simulink model "deadbeat_running_control"  (R2016b)
settings: configuration reference "Configuration1khz" (kept outside this file)
undefined symbols (not defined in the file or in its folder): A_kalman_no_position, A_kalman_transverse, A_kalman_vertical, A_lpf_accelerometer, A_lpf_contact, A_lpf_imu, A_lpf_lateral_angle, B1_lpf_accelerometer, B1_lpf_contact, B1_lpf_imu, B1_lpf_lateral_angle, B2_lpf_accelerometer, B2_lpf_contact, B2_lpf_imu, B2_lpf_lateral_angle, B_dx_versus_x0, B_kalman_no_position, B_kalman_transverse, B_kalman_vertical, backwards_K_sag_of_t, backwards_P_sag_of_t, C_kalman_no_position, C_kalman_transverse, C_kalman_vertical, com_leg_motor, com_torso, contact_threshold, d_ankle_to_foot, d_vertical_com, desired_com_forward_velocity, desired_com_lateral_velocity, desired_standing_torso_pitch, desired_standing_torso_roll, desired_standing_z, desired_torso_pitch, desired_torso_roll, DiscIntNeverNeededParam, Discrete, enable_bouncing, fdesignblkfcn, flight_duration, forward_dx_of_dxstar, forward_x_of_dxstar, g, gcbh, HIP_MTR_MAX_CONT_TORQUE, HIP_MTR_MAX_TORQUE, i_leg_motor, i_robot, i_torso, initial_dx_estimate, initial_dx_takeoff_history, initial_dx_touchdown_history, initial_dy_estimate, initial_dy_takeoff_history, initial_dy_touchdown_history, initial_dz_estimate, initial_leg_selection, initial_target_dx_history, initial_target_dy_history ... (+80)
libraries: simulink x22, ctrlSharedLib x4, dsparch4 x2
(part 4 of 7)

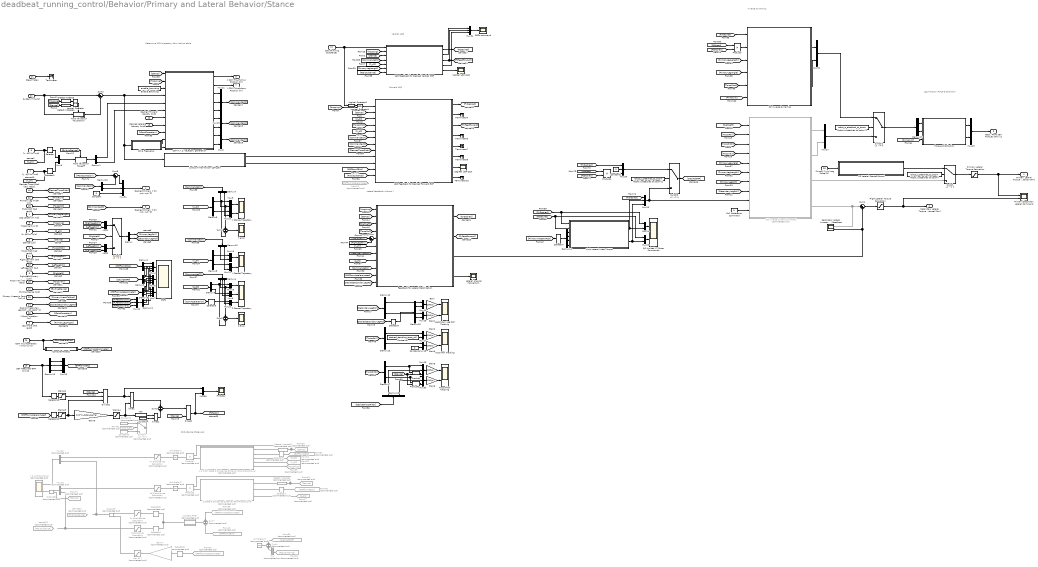
== system deadbeat_running_control/Behavior/Primary and Lateral Behavior/Stance ==
  note: Leg Torque / Force
      | Distribution
  note: Disturbance Observers
  note: Determine COM trajectory
      | from lookup table
  note: Forward LQR
  note: Inverse Dynamics
  note: Lateral feedback without Y
  note: Vertical LQR
  Leg Length [m m/s] : Inport
  Torso Pitch [rad rad/s] : Inport  Port=2
  Stance [1/0] : Inport  Port=3
  Leg Angle [rad rad/s] : Inport  Port=4
  Right/Left Primary [1/0] : Inport  Port=5
  "[x, dx] [m, m/s]" : Inport  Port=6
  "[y, dy] [m, m/s]" : Inport  Port=7
  "[z, dz] [m, m/s]" : Inport  Port=8
  Hopping [1 or 0] : Inport  Port=9
  SEA Measured GRF [N N N] : Inport  Port=10
  Steps Taken : Inport  Port=11
  Desired Forward Velocity [m/s] : Inport  Port=12
  Desired Lateral Velocity [m/s] : Inport  Port=13
  Right Leg Roll [rad rad/s] : Inport  Port=14
  Left Leg Roll [rad rad/s] : Inport  Port=15
  Torso Yaw [rad rad/s] : Inport  Port=16
  Exiting Stance [1/0] : Inport  Port=17
  "Desired Torso Pitch [rad, rad/s]" : Inport  Port=18
  Torso Roll [rad rad/s] : Inport  Port=19
  COM XYZ Acceleration [m/s^2] x3 : Inport  Port=20
  System Time [s] : Inport  Port=21
  Primary Leg Width [m] : Inport  Port=22
  Primary Knees to Foot [m] x6 : Inport  Port=23
  Desired Secondary Leg Roll [rad rad/s rad/s^2] : Inport  Port=24
  Primary Axial Leg Force [N] : Inport  Port=25
  X Foot Correction [m[ : Inport  Port=26
  Stop Running [true/false] : Inport  Port=27
  2D Inverse Dynamics : Subsystem
  2D Lateral Stance Control : MATLAB Function  TreatAsAtomicUnit=on
  3D Inverse Dynamics yawed : MATLAB Function  Commented=on  TreatAsAtomicUnit=on
  COM X,Y,Z  trajectory generation : MATLAB Function  TreatAsAtomicUnit=on
  Chirp Frequency : Subsystem
  Clamp2 : Saturate  UpperLimit=inf  LowerLimit=0
      settings: AttributesFormatString=Top: %<UpperLimit>\nBottom: %<LowerLimit>
  Clamp3 : Saturate  UpperLimit=inf  LowerLimit=1
      settings: AttributesFormatString=Top: %<UpperLimit>\nBottom: %<LowerLimit>
  Clamp4 : Saturate  UpperLimit=1  LowerLimit=0
      settings: AttributesFormatString=Top: %<UpperLimit>\nBottom: %<LowerLimit>
  Compute Forces1 : Subsystem
  Constant : Constant  Value=0
  Constant1 : Constant  Value=0
  Constant2 : Constant  Commented=on
  Constant3 : Constant  Value=desired_standing_torso_roll
  Constant4 : Constant  Value=0
  Constant5 : Constant  Commented=on  Value=0.87
  Constant6 : Constant
  Demux{,1,5,7..10,12..13,15,17..20} (14 alike) : Demux  Outputs=2
  Demux{2..4,6,11,16} (6 alike) : Demux  Outputs=3
  Demux14 : Demux
  Detect Increase : simulink/Logic and Bit Operations/Detect Increase  vinit=0.0  InputProcessing=Inherited  OutDataTypeStr=boolean
  Detect Increase1 : simulink/Logic and Bit Operations/Detect Increase  vinit=0.0  InputProcessing=Inherited  OutDataTypeStr=boolean
  Detect Increase2 : simulink/Logic and Bit Operations/Detect Increase  Commented=on  vinit=0.0  InputProcessing=Inherited  OutDataTypeStr=boolean
  Detect Increase3 : simulink/Logic and Bit Operations/Detect Increase  Commented=on  vinit=0.0  InputProcessing=Inherited  OutDataTypeStr=boolean
  "Disturbance Saturation " : Saturate  Commented=on  UpperLimit=100  LowerLimit=-100
      settings: AttributesFormatString=Top: %<UpperLimit>\nBottom: %<LowerLimit>
  Divide1 : Product  Inputs=**/
  Enable Bouncing : Constant  Value=enable_bouncing  SampleTime=sample_time
  Fcn : Fcn  Expr=1-u
  Feedback for Lateral Stabilization : MATLAB Function  TreatAsAtomicUnit=on
  Flight Lateral Torque Saturation : Saturate  UpperLimit=HIP_MTR_MAX_CONT_TORQUE  LowerLimit=-HIP_MTR_MAX_CONT_TORQUE
      settings: AttributesFormatString=Top: %<UpperLimit>\nBottom: %<LowerLimit>
  From10 : From  Commented=on  GotoTag=GRFfromAccelerometer
  From40 : From  Commented=on  GotoTag=GRFfromSEAs
  From47 : From  Commented=on  GotoTag=Z_dZ
  From48 : From  Commented=on  GotoTag=GRFfromSEAs
  From49 : From  Commented=on  GotoTag=Stance
  From50 : From  Commented=on  GotoTag=Stance
  From51 : From  Commented=on  GotoTag=GRFfromSEAs
  From52 : From  Commented=on  GotoTag=X_dX
  From53 : From  Commented=on  GotoTag=TorsoPitch
  From54 : From  Commented=on  GotoTag=Z_dZ
  From59 : From  Commented=on  GotoTag=GRFfromAccelerometer
  From61 : From  Commented=on  GotoTag=GRFfromAccelerometer
  From79 : From  Commented=on  GotoTag=Stance
  From80 : From  Commented=on  GotoTag=DesiredGRF
  From81 : From  Commented=on  GotoTag=FzDisturbance
  From82 : From  Commented=on  GotoTag=RightLeft
  Fx Disturbance Saturation : Saturate  Commented=on  UpperLimit=100  LowerLimit=-100
      settings: AttributesFormatString=Top: %<UpperLimit>\nBottom: %<LowerLimit>
  "Fx Disturbance Saturation " : Saturate  Commented=on  UpperLimit=30  LowerLimit=-30
      settings: AttributesFormatString=Top: %<UpperLimit>\nBottom: %<LowerLimit>
  Fz Disturbance Saturation : Saturate  Commented=on  UpperLimit=100  LowerLimit=-100
      settings: AttributesFormatString=Top: %<UpperLimit>\nBottom: %<LowerLimit>
  Fz Factor : Scope
  GRFs : Scope  NumInputPorts=3
  GRFz command : Scope
  Gain{,1..3,5..6} (6 alike) : Gain  Gain=180/pi
  Gain4 : Gain  Commented=on  Gain=2/(m_total_real*g)
  Gain8 : Gain  Gain=1/(2*m_total_real*g)
  Hold Values on Takeoff : Subsystem
  Hold Values on Touchdown : Subsystem
  LQR Feedback for Desired Forward GRF : MATLAB Function  TreatAsAtomicUnit=on
  LQR Feedback for Desired Vertical GRF : MATLAB Function  TreatAsAtomicUnit=on
  Lateral Angular Momentum : Scope
  Limit Lateral Knee Torque : MATLAB Function  TreatAsAtomicUnit=on
  Logical Operator : Logic  Operator=OR  AllPortsSameDT=off  OutDataTypeStr=boolean
  Logical Operator1 : Logic  AllPortsSameDT=off  OutDataTypeStr=boolean
  Logical Operator2 : Logic  Operator=NOT  AllPortsSameDT=off  OutDataTypeStr=boolean
  Lookup finite horizon LQR gain : MATLAB Function  TreatAsAtomicUnit=on
  Lowpass Filter : Subsystem  Commented=on  DialogController=fdesignblkfcn  InitFcn=fdesignblkfcn(gcbh, {'InitFcn'});  mask(Lowpass Filter){}
      mask help: Design a lowpass filter
      settings: CopyFcn=fdesignblkfcn(gcbh, {'CopyFcn'});
      mask Help: helpview(mapfilelocation('dsp'), 'dsplowpassfilter');
      mask Display: disp('Lowpass')
  Max of 1 : Saturate  Commented=on  UpperLimit=1  LowerLimit=0
      settings: AttributesFormatString=Top: %<UpperLimit>\nBottom: %<LowerLimit>
  Mux : Mux  Commented=on  Inputs=3
  Mux{1..3,5,8..10,12..18,22..25,27,32,35,49} (22 alike) : Mux  Inputs=2
  Mux{11,21,26,28..31,33..34} (9 alike) : Mux  Inputs=3
  Mux19 : Mux  Commented=on  Inputs=2
  Mux20 : Mux  Commented=on  Inputs=2
  Mux4 : Mux
  Mux6 : Mux
  Mux7 : Mux
  Primary Lateral Torque Saturation : Saturate  UpperLimit=max_primary_lateral_stance_torque  LowerLimit=-max_primary_lateral_stance_torque
      settings: AttributesFormatString=Top: %<UpperLimit>\nBottom: %<LowerLimit>
  Primary/Secondary Lateral Command : Scope  NumInputPorts=2
  Product{,4,6..7} (4 alike) : Product
  Product{1..3,5} (4 alike) : Product  Commented=on
  QP Limited YZ Force Commands : Scope  NumInputPorts=2
  Robot is attached to boom? : Constant  Value=robot_is_attached_to_boom
  Robot is attached to boom?1 : Constant  Value=robot_is_attached_to_boom
  Robot is attached to boom?2 : Constant  Value=robot_is_attached_to_boom
  Roll Accleration Command : Constant  Value=0
  Sagittal LQR Cost : Scope
  Secondary Lateral Inverse Dynamics / Feedback : Scope  NumInputPorts=2
  Secondary Leg Roll Tracking : Scope  NumInputPorts=2
  Selector : Selector  InputPortWidth=2  IndexOptions=Index vector (dialog)  Indices=[2]  OutputSizes=1
  Selector1 : Selector  InputPortWidth=2  IndexOptions=Index vector (dialog)  Indices=[2]  OutputSizes=1
  Selector10 : Selector  InputPortWidth=3  IndexOptions=Index vector (dialog)  Indices=[3]  OutputSizes=1
  Selector11 : Selector  InputPortWidth=3  IndexOptions=Index vector (dialog)  Indices=[3]  OutputSizes=1
  Selector2 : Selector  Commented=on  InputPortWidth=3  IndexOptions=Index vector (dialog)  Indices=[3]  OutputSizes=1
  Selector3 : Selector  Commented=on  InputPortWidth=3  IndexOptions=Index vector (dialog)  Indices=[1]  OutputSizes=1
  Selector4 : Selector  Commented=on  InputPortWidth=3  IndexOptions=Index vector (dialog)  Indices=[3]  OutputSizes=1
  Selector5 : Selector  Commented=on  InputPortWidth=3  IndexOptions=Index vector (dialog)  Indices=[1]  OutputSizes=1
  Selector6 : Selector  InputPortWidth=3  IndexOptions=Index vector (dialog)  Indices=[3]  OutputSizes=1
  Selector7 : Selector  InputPortWidth=6  IndexOptions=Index vector (dialog)  Indices=[2 5 3 6]  OutputSizes=1
  Selector8 : Selector  Commented=on  InputPortWidth=3  IndexOptions=Index vector (dialog)  Indices=[3]  OutputSizes=1
  Selector9 : Selector  InputPortWidth=3  IndexOptions=Index vector (dialog)  Indices=[1 2]  OutputSizes=1
  Sum : Sum  Inputs=|+-
  Sum1 : Sum  Commented=on
  Sum2 : Sum  Inputs=|+-
  Sum3 : Sum  Inputs=+|+
  Sum4 : Sum  Inputs=|++
  Sum5 : Sum  Inputs=+-
  Sum6 : Sum  Inputs=+-
  Sum7 : Sum  Commented=on  Inputs=+-
  Sum8 : Sum  Inputs=|++
  Switch{,1..3} (4 alike) : Switch  Criteria=u2 ~= 0
  Switch4 : Switch  Commented=on  Criteria=u2 ~= 0
  Terminator{,4,6..8,10} (6 alike) : Terminator
  Torque Distribution : Subsystem
  Torso Pitch Tracking : Scope  NumInputPorts=2
  Torso Roll Tracking : Scope  NumInputPorts=2
  Unit Delay1 : UnitDelay  Commented=on  SampleTime=sample_time
  Unit Delay2 : UnitDelay  Commented=on  SampleTime=sample_time
  Unit Delay3 : UnitDelay  Commented=on  SampleTime=sample_time
  Vertical LQR Cost : Scope
  X & Pitch State Disturbance Observer Error-Proportional : MATLAB Function  Commented=on  TreatAsAtomicUnit=on
  X & Z Disturbance : Scope  Commented=on  NumInputPorts=2
  X Stance Trajectory : Scope  NumInputPorts=2
  X error : Scope
  Y Stance Trajectory : Scope  NumInputPorts=2
  Z Error : Scope
  Z Stance Trajectory : Scope  NumInputPorts=3
  Z State Disturbance Observer Error-Proportional : MATLAB Function  Commented=on  TreatAsAtomicUnit=on
  stance21 : Goto  Commented=on  GotoTag=FxDisturbance
  stance22 : Goto  Commented=on  GotoTag=FzDisturbance
  times : Product  Inputs=**
  times1 : Product  Inputs=**
  times2 : Product  Inputs=**
  Primary Lateral Torque Command (stance) [Nm] : Outport
  Secondary Lateral Torque Command (stance) [Nm] : Outport  Port=2
  Back / Front SEA Torques [Nm] x2 : Outport  Port=3
  "Desired Primary X [m, m/s, m/s^2]" : Outport  Port=4
  "Desired Primary Z [m, m/s, m/s^2]" : Outport  Port=5
  X COM Touchdown Position [m] : Outport  Port=6
  Y COM Touchdown Position [m] : Outport  Port=7
  wires:
  "Disturbance Saturation "/1 -> Mux19/2
  Sum1/1 -> Unit Delay3/1
  Mux/1 -> Sum1/2
  From81/1 -> Mux/3
  From80/1 -> Sum1/1
  Selector9/1 -> Demux15/1
  Lowpass Filter/1(Out) -> Selector4/1, Selector5/1
  Sum7/1 -> Lowpass Filter/1(In)
  From79/1 -> Product5/2
  Mux19/1 -> Product5/1
  Limit Lateral Knee Torque/1(Fy_command) -> Mux26/2, Mux24/2
  Mux25/1 -> QP Limited YZ Force Commands/2
  Mux24/1 -> QP Limited YZ Force Commands/1
  Selector7/1 -> Demux14/1
  Demux14/4 -> Limit Lateral Knee Torque/6(z_knee_back)
  Demux14/3 -> Limit Lateral Knee Torque/5(z_knee_front)
  Demux14/2 -> Limit Lateral Knee Torque/4(y_knee_back)
  Demux14/1 -> Limit Lateral Knee Torque/3(y_knee_front)
  [PrimaryKneesToFoot] -> Selector7/1
  Primary Knees to Foot [m] x6/1 -> [PrimaryKneesToFoot]
  Feedback for Lateral Stabilization/2(neutral_feedforward_Fy) -> [FyFeedforward]
  LQR Feedback for Desired Forward GRF/2(netural_ff) -> Terminator4/1
  LQR Feedback for Desired Forward GRF/3(true_ff) -> [FxFeedforward]
  Compute Forces1/1(XYZ Force) -> [GRFfromAccelerometer]
  [FyFeedforward] -> Mux21/2
  [Z_dZ] -> Feedback for Lateral Stabilization/8(z_dz)
  [FzDesired] -> Mux25/1, Limit Lateral Knee Torque/2(Fz_s)
  [FxFeedforward] -> Mux21/1
  Mux23/1 -> Back / Front SEA Torques [Nm] x2/1
  Torque Distribution/2(Front Torque [Nm]) -> Mux23/2
  Torque Distribution/1(Back Torque [Nm]) -> Mux23/1
  Primary Leg Width [m]/1 -> [PrimaryW]
  3D Inverse Dynamics yawed/2(primary_leg_force) -> Mux27/2
  [PrimaryW] -> Torque Distribution/3(w [m])
  3D Inverse Dynamics yawed/1(primary_leg_torque) -> Mux27/1
  Selector6/1 -> Mux22/1
  [ComAcceleration] -> Selector6/1
  Mux22/1 -> Z Stance Trajectory/3
  Sum5/1 -> Z Error/1
  [CommandedZ] -> Demux4/1
  Demux4/3 -> Mux22/2
  Demux4/2 -> Mux8/2
  Demux4/1 -> Sum5/1, Mux15/2
  Demux9/2 -> Mux8/1
  Demux9/1 -> Sum5/2, Mux15/1
  [Z_dZ] -> Demux9/1
  Mux8/1 -> Z Stance Trajectory/2
  Mux15/1 -> Z Stance Trajectory/1
  [FzFeedforward] -> Mux21/3
  Mux21/1 -> Demux11/1
  [GRFfromAccelerometer] -> Demux6/1
  COM XYZ Acceleration [m/s^2] x3/1 -> [ComAcceleration], Compute Forces1/1(XYZ Acceleration)
  From40/1 -> Sum7/2
  Product5/1 -> X & Z Disturbance/2
  From49/1 -> Detect Increase2/1, Product2/1
  Z State Disturbance Observer Error-Proportional/1(d_hat_tp1) -> Product2/2
  From50/1 -> Detect Increase3/1, Product1/1
  X & Pitch State Disturbance Observer Error-Proportional/1(d_hat_tp1) -> Product1/2
  Product2/1 -> Unit Delay2/1
  Product1/1 -> Unit Delay1/1
  From47/1 -> Z State Disturbance Observer Error-Proportional/3(z_dz)
  From48/1 -> Selector2/1
  Detect Increase2/1 -> Z State Disturbance Observer Error-Proportional/1(enabled)
  Detect Increase3/1 -> X & Pitch State Disturbance Observer Error-Proportional/1(enabled)
  From51/1 -> Selector3/1
  From52/1 -> X & Pitch State Disturbance Observer Error-Proportional/4(x_dx)
  From53/1 -> X & Pitch State Disturbance Observer Error-Proportional/5(theta_dtheta)
  From54/1 -> X & Pitch State Disturbance Observer Error-Proportional/3(z_dz)
  "[z, dz] [m, m/s]"/1 -> [Z_dZ]
  Flight Lateral Torque Saturation/1 -> Secondary Lateral Torque Command (stance) [Nm]/1, Primary/Secondary Lateral Command/2
  Demux6/3 -> Mux7/3
  Demux6/2 -> Mux6/3
  Demux6/1 -> Mux4/3
  Feedback for Lateral Stabilization/4(angular_momentum) -> Lateral Angular Momentum/1
  LQR Feedback for Desired Forward GRF/4(GRFx_lqr) -> Terminator6/1
  [Stance] -> COM X,Y,Z  trajectory generation/1(stance)
  Lookup finite horizon LQR gain/2(P_sag) -> LQR Feedback for Desired Forward GRF/10(P_sag)
  COM X,Y,Z  trajectory generation/3(z_ref) -> Mux11/1
  [Stance] -> LQR Feedback for Desired Forward GRF/2(stance)
  COM X,Y,Z  trajectory generation/6(x_ref) -> Mux49/1
  COM X,Y,Z  trajectory generation/7(dx_ref) -> Mux49/2
  COM X,Y,Z  trajectory generation/8(y_ref) -> Mux5/1
  COM X,Y,Z  trajectory generation/9(dy_ref) -> Mux5/2
  COM X,Y,Z  trajectory generation/1(x_0) -> X COM Touchdown Position [m]/1
  COM X,Y,Z  trajectory generation/4(dz_ref) -> Mux11/2
  COM X,Y,Z  trajectory generation/5(ddz_ref) -> Mux11/3
  Mux11/1 -> [CommandedZ]
  [X_dX] -> LQR Feedback for Desired Forward GRF/3(xdx)
  [TorsoPitch] -> LQR Feedback for Desired Forward GRF/4(thetadtheta)
  [DesiredTorsoPitch] -> LQR Feedback for Desired Forward GRF/8(thetadtheta_star)
  Lookup finite horizon LQR gain/1(K_sag) -> LQR Feedback for Desired Forward GRF/9(K_sag)
  [Z_dZ] -> LQR Feedback for Desired Forward GRF/5(zdz)
  Desired Forward Velocity [m/s]/1 -> COM X,Y,Z  trajectory generation/7(target_DX)
  Sum2/1 -> COM X,Y,Z  trajectory generation/4(t), Lookup finite horizon LQR gain/1(t_forward), Chirp Frequency/1(Time Since Stance)
  Hold Values on Touchdown/1(out) -> Sum2/2
  Stance [1/0]/1 -> [Stance]
  Logical Operator/1 -> Hold Values on Touchdown/Trigger
  "[x, dx] [m, m/s]"/1 -> [X_dX], Selector/1
  Demux1/2 -> COM X,Y,Z  trajectory generation/6(dy0)
  LQR Feedback for Desired Forward GRF/5(ddtheta_star) -> Terminator7/1
  LQR Feedback for Desired Forward GRF/6(ddtheta_star_neutral) -> Terminator8/1
  LQR Feedback for Desired Forward GRF/7(cost_to_go) -> Sagittal LQR Cost/1
  LQR Feedback for Desired Forward GRF/8(ang_mom) -> Terminator10/1
  Torso Pitch [rad rad/s]/1 -> [TorsoPitch]
  [RightLeft] -> 3D Inverse Dynamics yawed/1(right_or_left)
  Hopping [1 or 0]/1 -> [Hopping]
  [Hopping] -> COM X,Y,Z  trajectory generation/2(hopping)
  [GRFfromSEAs] -> LQR Feedback for Desired Forward GRF/11(measured_GRF)
  Steps Taken/1 -> Terminator/1
  Detect Increase/1 -> Logical Operator/1
  Detect Increase1/1 -> Logical Operator/2
  [Hopping] -> Detect Increase/1
  [Stance] -> Detect Increase1/1
  Demux1/1 -> COM X,Y,Z  trajectory generation/5(dx0)
  Selector/1 -> Mux3/1
  [Stance] -> Feedback for Lateral Stabilization/2(stance)
  [TorsoRoll] -> Feedback for Lateral Stabilization/4(rolldroll)
  COM X,Y,Z  trajectory generation/2(y_0) -> Y COM Touchdown Position [m]/1
  Mux5/1 -> [CommandedY]
  [TorsoPitch] -> 3D Inverse Dynamics yawed/3(torso_pitch)
  [TorsoRoll] -> 3D Inverse Dynamics yawed/2(torso_roll)
  [TorsoYaw] -> 3D Inverse Dynamics yawed/4(torso_yaw)
  [PrimaryLegLength] -> 3D Inverse Dynamics yawed/6(primary_leg_length)
  [PrimaryLegAngle] -> 3D Inverse Dynamics yawed/5(primary_sagittal_leg_angle)
  [SecondaryLegRoll] -> 3D Inverse Dynamics yawed/8(secondary_leg_roll)
  [PrimaryLegRoll] -> 3D Inverse Dynamics yawed/7(primary_leg_roll)
  Switch1/1 -> Demux/1
  Demux/2 -> [SecondaryLegRoll]
  Demux/1 -> [PrimaryLegRoll]
  Mux1/1 -> Switch1/1
  Mux2/1 -> Switch1/3
  Right Leg Roll [rad rad/s]/1 -> [RightLegRoll]
  [RightLegRoll] -> Mux1/1
  [LeftLegRoll] -> Mux1/2
  [LeftLegRoll] -> Mux2/1
  [RightLegRoll] -> Mux2/2
  [RightLeft] -> Switch1/2
  "[y, dy] [m, m/s]"/1 -> [Y_dY], Selector1/1
  Mux3/1 -> Hold Values on Takeoff/1(in)
  Hold Values on Takeoff/1(out) -> Demux1/1
  Selector1/1 -> Mux3/2
  Desired Lateral Velocity [m/s]/1 -> COM X,Y,Z  trajectory generation/8(target_DY)
  Torso Yaw [rad rad/s]/1 -> [TorsoYaw]
  Exiting Stance [1/0]/1 -> [ExitingStance]
  [ExitingStance] -> Hold Values on Takeoff/Trigger
  [Hopping] -> Feedback for Lateral Stabilization/1(hopping)
  [GRFfromAccelerometer] -> Feedback for Lateral Stabilization/10(GRF_measured)
  System Time [s]/1 -> Hold Values on Touchdown/1(in), Sum2/1
  Leg Length [m m/s]/1 -> [PrimaryLegLength]
  Torso Roll [rad rad/s]/1 -> [TorsoRoll]
  [GRFfromSEAs] -> Demux2/1
  [DesiredGRF] -> Demux3/1
  Mux4/1 -> GRFs/1
  Demux2/1 -> Mux4/1
  Mux6/1 -> GRFs/2
  Mux7/1 -> GRFs/3
  Demux2/2 -> Mux6/1
  Demux2/3 -> Mux7/1
  Demux3/1 -> Mux4/2
  Demux3/2 -> Mux6/2
  Demux3/3 -> Mux7/2
  Mux9/1 -> X Stance Trajectory/1
  Mux10/1 -> X Stance Trajectory/2
  Demux5/2 -> Mux10/1
  Demux7/2 -> Mux10/2
  [X_dX] -> Demux5/1
  Mux13/1 -> Y Stance Trajectory/1
  Mux12/1 -> Y Stance Trajectory/2
  Demux8/1 -> Mux13/1
  Demux8/2 -> Mux12/1
  Demux10/1 -> Mux13/2
  Demux10/2 -> Mux12/2
  [Y_dY] -> Demux8/1
  [CommandedX] -> Demux7/1
  [CommandedY] -> Demux10/1
  Right/Left Primary [1/0]/1 -> [RightLeft]
  Left Leg Roll [rad rad/s]/1 -> [LeftLegRoll]
  LQR Feedback for Desired Forward GRF/1(GRFx_desired) -> [FxDesired]
  Demux11/1 -> Mux4/4
  Demux11/2 -> Mux6/4
  Demux11/3 -> Mux7/4
  Primary Lateral Torque Saturation/1 -> Primary Lateral Torque Command (stance) [Nm]/1, Primary/Secondary Lateral Command/1
  [FyDesired] -> Mux24/1, Limit Lateral Knee Torque/1(Fy_s)
  Roll Accleration Command/1 -> 3D Inverse Dynamics yawed/10(ddRoll_desired)
  [LeftLegRoll] -> Sum/1
  [RightLegRoll] -> Sum/2
  [Y_dY] -> Feedback for Lateral Stabilization/6(y_dy)
  [SecondaryLegRoll] -> Feedback for Lateral Stabilization/7(beta2dbeta2)
  Sum/1 -> Feedback for Lateral Stabilization/5(symdsym)
  3D Inverse Dynamics yawed/4(secondary_lateral_torque) -> Sum4/1, Secondary Lateral Inverse Dynamics / Feedback/1
  Switch/1 -> Primary Lateral Torque Saturation/1
  Sum4/1 -> Flight Lateral Torque Saturation/1
  Feedback for Lateral Stabilization/3(secondary_lateral_torque_desired) -> Secondary Lateral Inverse Dynamics / Feedback/2, Sum4/2
  [TorsoRoll] -> Demux13/1
  Gain2/1 -> Torso Roll Tracking/1
  Gain3/1 -> Torso Roll Tracking/2
  Mux17/1 -> Gain2/1
  Demux13/1 -> Mux17/1
  Constant3/1 -> Mux17/2
  Demux13/2 -> Mux18/1
  Mux18/1 -> Gain3/1
  Constant4/1 -> Mux18/2
  [RightLeft] -> Feedback for Lateral Stabilization/3(right_left)
  Enable Bouncing/1 -> COM X,Y,Z  trajectory generation/3(bouncing)
  Fx Disturbance Saturation/1 -> Mux20/1
  Selector3/1 -> X & Pitch State Disturbance Observer Error-Proportional/2(Fx)
  Unit Delay1/1 -> Fx Disturbance Saturation/1
  Unit Delay2/1 -> Fz Disturbance Saturation/1
  Demux5/1 -> Sum6/2, Mux9/1
  Demux7/1 -> Sum6/1, Mux9/2
  Sum6/1 -> X error/1
  From59/1 -> Sum7/1
  Mux20/1 -> X & Z Disturbance/1
  Product3/1 -> Mux20/2
  Selector2/1 -> Z State Disturbance Observer Error-Proportional/2(Fz)
  Chirp Frequency/1(w) -> COM X,Y,Z  trajectory generation/10(standing_bounce_w)
  Chirp Frequency/2(dw/dt) -> COM X,Y,Z  trajectory generation/11(standing_bounce_dw)
  [FxDisturbance] -> LQR Feedback for Desired Forward GRF/12(Fx_disturbance)
  Limit Lateral Knee Torque/2(Fz_command) -> Mux26/3, Mux25/2
  From61/1 -> Selector8/1
  Selector8/1 -> Gain4/1
  Gain4/1 -> Max of 1/1
  "Fx Disturbance Saturation "/1 -> Product3/1
  Max of 1/1 -> Product3/2
  Selector4/1 -> "Disturbance Saturation "/1
  Selector5/1 -> "Fx Disturbance Saturation "/1
  Fz Disturbance Saturation/1 -> Mux19/1
  [DesiredSecondaryLegRoll] -> Feedback for Lateral Stabilization/11(desired_beta2_state)
  Desired Secondary Leg Roll [rad rad/s rad/s^2]/1 -> [DesiredSecondaryLegRoll]
  Primary Axial Leg Force [N]/1 -> 2D Lateral Stance Control/1(F_leg)
  2D Lateral Stance Control/1(lateral_torque) -> Switch/1
  Robot is attached to boom?/1 -> Switch/2
  3D Inverse Dynamics yawed/3(primary_lateral_torque) -> Switch/3
  Feedback for Lateral Stabilization/1(Fy_desired) -> [FyDesired]
  Robot is attached to boom?1/1 -> Switch2/2
  Mux32/1 -> Switch2/1
  [FxDesired] -> Mux26/1
  Demux15/2 -> Mux16/2
  Demux12/2 -> Mux16/1
  Mux16/1 -> Gain1/1
  Gain1/1 -> Secondary Leg Roll Tracking/2
  Gain/1 -> Secondary Leg Roll Tracking/1
  Demux15/1 -> Mux14/2
  Demux12/1 -> Mux14/1
  Mux14/1 -> Gain/1
  [SecondaryLegRoll] -> Demux12/1
  [DesiredSecondaryLegRoll] -> Selector9/1
  [TorsoPitch] -> Demux17/1
  Gain5/1 -> Torso Pitch Tracking/1
  Gain6/1 -> Torso Pitch Tracking/2
  Mux29/1 -> Gain5/1
  Demux17/1 -> Product/1, Mux29/1
  Demux18/1 -> Mux29/2
  Demux17/2 -> Product6/1, Mux30/1
  Mux30/1 -> Gain6/1
  Demux18/2 -> Mux30/2
  "Desired Torso Pitch [rad, rad/s]"/1 -> [DesiredTorsoPitch]
  [CommandedX] -> LQR Feedback for Desired Forward GRF/6(xdx_ref)
  [CommandedZ] -> LQR Feedback for Desired Forward GRF/7(zdzddz_ref)
  [CommandedZ] -> Feedback for Lateral Stabilization/9(zdzddz_ref)
  [DesiredTorsoPitch] -> Demux18/1
  Mux49/1 -> [CommandedX]
  Constant/1 -> Mux31/3
  [CommandedZ] -> "Desired Primary Z [m, m/s, m/s^2]"/1
  X Foot Correction [m[/1 -> [XFootCorrection]
  Product/1 -> Mux29/3
  Product6/1 -> Mux30/3
  [Stance] -> Product6/2, Product/2
  [XFootCorrection] -> COM X,Y,Z  trajectory generation/9(x_foot_correction)
  [FzDesired] -> Product7/2
  [FzFactor] -> Product7/1
  [FxDesired] -> 2D Inverse Dynamics/1(Fx Desired [N])
  [PrimaryLegLength] -> 2D Inverse Dynamics/3(Leg Length [m m/s])
  Leg Angle [rad rad/s]/1 -> [PrimaryLegAngle]
  [PrimaryLegAngle] -> 2D Inverse Dynamics/4(Leg Angle [rad rad/s])
  [TorsoPitch] -> 2D Inverse Dynamics/5(Torso Pitch [rad rad/s])
  [PrimaryW] -> 2D Inverse Dynamics/6(Primary w [m])
  2D Inverse Dynamics/1(Leg Torque [Nm]) -> Mux32/1
  2D Inverse Dynamics/2(Leg Force [N]) -> Mux32/2
  Mux27/1 -> Switch2/3
  Demux19/1 -> Torque Distribution/1(Leg Torque [Nm])
  Demux19/2 -> Torque Distribution/2(Leg Force [N])
  Switch2/1 -> Demux19/1
  Robot is attached to boom?2/1 -> Switch3/2
  Mux26/1 -> 3D Inverse Dynamics yawed/9(GRF_desired), Switch3/3
  Switch3/1 -> [DesiredGRF]
  [FzDesired] -> Product4/2
  [FzFactor] -> Product4/1
  [FxDesired] -> Mux33/1
  Product4/1 -> Mux33/3
  Mux33/1 -> Switch3/1
  Constant1/1 -> Mux33/2
  Product7/1 -> 2D Inverse Dynamics/2(Fz Desired [N])
  [CommandedZ] -> LQR Feedback for Desired Vertical GRF/4(zdzddz_ref)
  [FzDisturbance] -> LQR Feedback for Desired Vertical GRF/7(Fz_disturbance)
  [PrimaryLegLength] -> LQR Feedback for Desired Vertical GRF/6(leg_length)
  [Hopping] -> LQR Feedback for Desired Vertical GRF/2(hopping)
  LQR Feedback for Desired Vertical GRF/5(cost_to_go) -> Vertical LQR Cost/1
  [Stance] -> LQR Feedback for Desired Vertical GRF/3(stance)
  LQR Feedback for Desired Vertical GRF/1(GRFz_desired) -> [FzDesired]
  [Z_dZ] -> LQR Feedback for Desired Vertical GRF/5(z_state)
  LQR Feedback for Desired Vertical GRF/3(GRFz_feedforward) -> Mux34/2, [FzFeedforward]
  Mux34/1 -> GRFz command/1
  LQR Feedback for Desired Vertical GRF/2(GRFz_feedback) -> Mux34/1
  LQR Feedback for Desired Vertical GRF/4(GRFz_integral) -> Mux34/3
  Mux28/1 -> [GRFfromSEAs]
  Demux16/2 -> Mux28/2
  SEA Measured GRF [N N N]/1 -> Selector10/1, Demux16/1
  [GRFfromAccelerometer] -> Selector11/1
  Selector10/1 -> Clamp2/1
  Selector11/1 -> Clamp3/1
  Demux16/3 -> Mux28/3
  [Stance] -> Divide1/1
  Clamp2/1 -> Divide1/2
  Clamp3/1 -> Gain8/1, Divide1/3
  Divide1/1 -> Mux35/1, times/1
  times2/1 -> Mux35/2, [FzFactor]
  Gain8/1 -> Clamp4/1
  Clamp4/1 -> times/2, Fcn/1
  times/1 -> Sum3/1
  Fcn/1 -> times1/1
  Constant6/1 -> times1/2
  times1/1 -> Sum3/2
  Sum3/1 -> times2/1
  [Stance] -> times2/2
  Mux35/1 -> Fz Factor/1
  Constant5/1 -> Switch4/3
  Constant2/1 -> Switch4/1
  From82/1 -> Switch4/2
  Demux16/1 -> Mux28/1
  Mux31/1 -> "Desired Primary X [m, m/s, m/s^2]"/1
  [CommandedX] -> Demux20/1
  Demux20/2 -> Mux31/2
  [XFootCorrection] -> Sum8/1
  Demux20/1 -> Sum8/2
  Sum8/1 -> Mux31/1
  Stop Running [true/false]/1 -> LQR Feedback for Desired Vertical GRF/1(stop_running), Logical Operator2/1
  Logical Operator1/1 -> LQR Feedback for Desired Forward GRF/1(hopping)
  [Hopping] -> Logical Operator1/2
  Logical Operator2/1 -> Logical Operator1/1

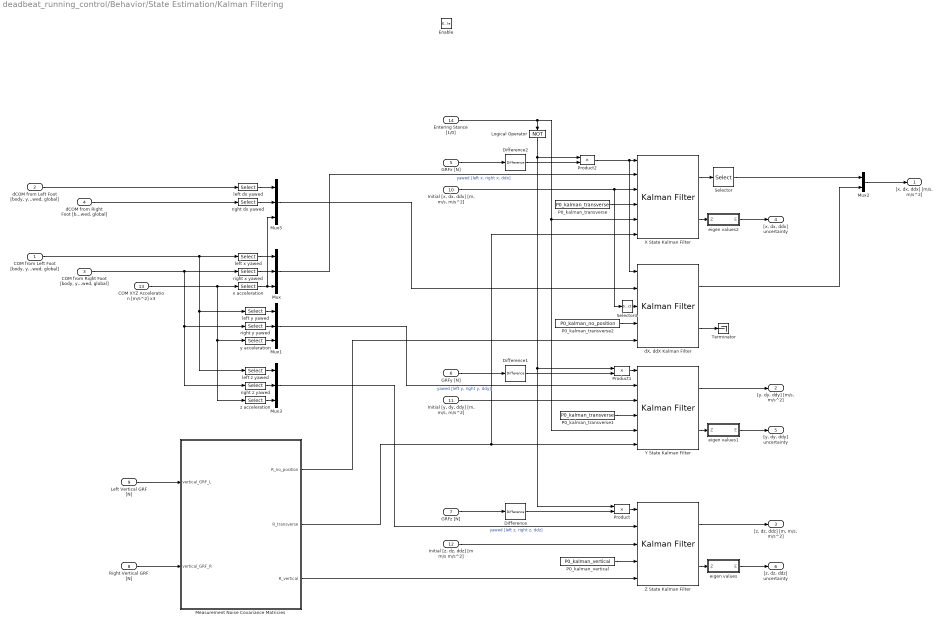
== system deadbeat_running_control/Behavior/State Estimation/Kalman Filtering ==
  "COM from Left Foot [body, yawed, global]" : Inport  SampleTime=sample_time
  "dCOM from Left Foot [body, yawed, global]" : Inport  Port=2  SampleTime=sample_time
  "COM from Right Foot [body, yawed, global]" : Inport  Port=3  SampleTime=sample_time
  "dCOM from Right Foot [body, yawed, global]" : Inport  Port=4  SampleTime=sample_time
  GRFx [N] : Inport  Port=5  SampleTime=sample_time
  GRFy [N] : Inport  Port=6  SampleTime=sample_time
  GRFz [N] : Inport  Port=7  SampleTime=sample_time
  Right Vertical GRF [N] : Inport  Port=8  SampleTime=sample_time
  Left Vertical GRF [N] : Inport  Port=9  SampleTime=sample_time
  "Initial [x, dx, ddx] [m, m/s, m/s^2]" : Inport  Port=10  PortDimensions=3  SampleTime=sample_time
  "Initial [y, dy, ddy] [m, m/s, m/s^2]" : Inport  Port=11  PortDimensions=3  SampleTime=sample_time
  "Initial [z, dz, ddz] [m m/s m/s^2]" : Inport  Port=12  PortDimensions=3  SampleTime=sample_time
  COM XYZ Acceleration [m/s^2] x3 : Inport  Port=13  SampleTime=sample_time
  Entering Stance [1/0] : Inport  Port=14  PortDimensions=1  SampleTime=sample_time
  Enable : EnablePort  StatesWhenEnabling=reset
  Difference : simulink/Discrete/Difference  ICPrevInput=0.0  InputProcessing=Inherited  OutMin=[]  OutMax=[]  OutDataType=fixdt(1, 16)  OutScaling=2^-10  DoSatur=off
  Difference1 : simulink/Discrete/Difference  ICPrevInput=0.0  InputProcessing=Inherited  OutMin=[]  OutMax=[]  OutDataType=fixdt(1, 16)  OutScaling=2^-10  DoSatur=off
  Difference2 : simulink/Discrete/Difference  ICPrevInput=0.0  InputProcessing=Inherited  OutMin=[]  OutMax=[]  OutDataType=fixdt(1, 16)  OutScaling=2^-10  DoSatur=off
  Logical Operator : Logic  Operator=NOT  AllPortsSameDT=off  OutDataTypeStr=boolean
  Measurement Noise Covariance Matricies : MATLAB Function  TreatAsAtomicUnit=on
  Mux{,1,3,5} (4 alike) : Mux  Inputs=3
  Mux2 : Mux  Inputs=2
  P0_kalman_transverse : Constant  Value=P0_kalman_transverse
  P0_kalman_transverse1 : Constant  Value=P0_kalman_transverse
  P0_kalman_transverse2 : Constant  Value=P0_kalman_no_position
  P0_kalman_vertical : Constant  Value=P0_kalman_vertical
  Product : Product
  Product1 : Product
  Product2 : Product
  Selector : Selector  InputPortWidth=3  IndexOptions=Index vector (dialog)  Indices=[1]  OutputSizes=1
  Selector4 : Selector  InputPortWidth=3  IndexOptions=Index vector (dialog)  Indices=[2 3]  OutputSizes=1
  Terminator : Terminator
  X State Kalman Filter : ctrlSharedLib/Kalman Filter  TimeDomain=Discrete-Time  UseCurrentEstimator=on  ModelSource=Individual A, B, C, D matrices  ModelSourceVariable=A_kf  A=A_kalman_transverse  B=B_kalman_transverse  C=C_kalman_transverse  D=0  NumberOfStates=2  NumberOfInputs=1  NumberOfOutputs=2  InitialEstimateSource=Input port  X0=initial_dx_estimate  P0=P0_kalman_transverse  UseK=off  UseGH=on  NumberOfProcessNoiseInputs=1  G=G_kalman_transverse  TimeInvariantG=on  H=0  TimeInvariantH=on  Q=Q_kalman_GRFx_difference*sample_time  TimeInvariantQ=on  R=1  TimeInvariantR=off  N=0  TimeInvariantN=on  AddInputPort=on  AddEnablePort=off  ExternalReset=Rising  OutputEstimatedY=off  OutputP=on  Ts=sample_time
  Y State Kalman Filter : ctrlSharedLib/Kalman Filter  TimeDomain=Discrete-Time  UseCurrentEstimator=on  ModelSource=Individual A, B, C, D matrices  ModelSourceVariable=A_kf  A=A_kalman_transverse  B=B_kalman_transverse  C=C_kalman_transverse  D=0  NumberOfStates=2  NumberOfInputs=1  NumberOfOutputs=2  InitialEstimateSource=Input port  X0=initial_dy_estimate  P0=P0_kalman_transverse  UseK=off  UseGH=on  NumberOfProcessNoiseInputs=1  G=G_kalman_transverse  TimeInvariantG=on  H=0  TimeInvariantH=on  Q=Q_kalman_GRFy_difference*sample_time  TimeInvariantQ=on  R=1  TimeInvariantR=off  N=0  TimeInvariantN=on  AddInputPort=on  AddEnablePort=off  ExternalReset=Rising  OutputEstimatedY=off  OutputP=on  Ts=sample_time
  Z State Kalman Filter : ctrlSharedLib/Kalman Filter  TimeDomain=Discrete-Time  UseCurrentEstimator=on  ModelSource=Individual A, B, C, D matrices  ModelSourceVariable=A_kf  A=A_kalman_vertical  B=B_kalman_vertical  C=C_kalman_vertical  D=0  NumberOfStates=2  NumberOfInputs=1  NumberOfOutputs=2  InitialEstimateSource=Input port  X0=[initial_z_estimate; initial_dz_estimate]  P0=P0_kalman_vertical  UseK=off  UseGH=on  NumberOfProcessNoiseInputs=1  G=G_kalman_vertical  TimeInvariantG=on  H=0  TimeInvariantH=on  Q=Q_kalman_GRFz_difference*sample_time  TimeInvariantQ=on  R=1  TimeInvariantR=off  N=0  TimeInvariantN=on  AddInputPort=on  AddEnablePort=off  OutputEstimatedY=off  OutputP=on  Ts=sample_time
  "dX, ddX Kalman Filter" : ctrlSharedLib/Kalman Filter  TimeDomain=Discrete-Time  UseCurrentEstimator=on  ModelSource=Individual A, B, C, D matrices  ModelSourceVariable=A_kf  A=A_kalman_no_position  B=B_kalman_no_position  C=C_kalman_no_position  D=0  NumberOfStates=2  NumberOfInputs=1  NumberOfOutputs=2  InitialEstimateSource=Input port  X0=initial_dx_estimate  P0=P0_kalman_transverse  UseK=off  UseGH=on  NumberOfProcessNoiseInputs=1  G=G_kalman_no_position  TimeInvariantG=on  H=0  TimeInvariantH=on  Q=Q_kalman_GRFx_difference*sample_time  TimeInvariantQ=on  R=1  TimeInvariantR=off  N=0  TimeInvariantN=on  AddInputPort=on  AddEnablePort=off  OutputEstimatedY=off  OutputP=on  Ts=sample_time
  eigen values : MATLAB Function  TreatAsAtomicUnit=on
  eigen values1 : MATLAB Function  TreatAsAtomicUnit=on
  eigen values2 : MATLAB Function  TreatAsAtomicUnit=on
  left dx yawed : Selector  InputPortWidth=9  IndexOptions=Index vector (dialog)  Indices=[4]  OutputSizes=1
  left x yawed : Selector  InputPortWidth=9  IndexOptions=Index vector (dialog)  Indices=[4]  OutputSizes=1
  left y yawed : Selector  InputPortWidth=9  IndexOptions=Index vector (dialog)  Indices=[5]  OutputSizes=1
  left z yawed : Selector  InputPortWidth=9  IndexOptions=Index vector (dialog)  Indices=[6]  OutputSizes=1
  right dx yawed : Selector  InputPortWidth=9  IndexOptions=Index vector (dialog)  Indices=[4]  OutputSizes=1
  right x yawed : Selector  InputPortWidth=9  IndexOptions=Index vector (dialog)  Indices=[4]  OutputSizes=1
  right y yawed : Selector  InputPortWidth=9  IndexOptions=Index vector (dialog)  Indices=[5]  OutputSizes=1
  right z yawed : Selector  InputPortWidth=9  IndexOptions=Index vector (dialog)  Indices=[6]  OutputSizes=1
  x acceleration : Selector  InputPortWidth=3  IndexOptions=Index vector (dialog)  Indices=[1]  OutputSizes=1
  y acceleration : Selector  InputPortWidth=3  IndexOptions=Index vector (dialog)  Indices=[2]  OutputSizes=1
  z acceleration : Selector  InputPortWidth=3  IndexOptions=Index vector (dialog)  Indices=[3]  OutputSizes=1
  "[x, dx, ddx] [m/s, m/s^2]" : Outport
  "[y, dy, ddy] [m/s, m/s^2]" : Outport  Port=2
  "[z, dz, ddz] [m, m/s, m/s^2]" : Outport  Port=3
  "[x, dx, ddx] uncertainty" : Outport  Port=4
  "[y, dy, ddy] uncertainty" : Outport  Port=5
  "[z, dz, ddz] uncertainty" : Outport  Port=6
  wires:
  "dCOM from Right Foot [body, yawed, global]"/1 -> right dx yawed/1
  "dCOM from Left Foot [body, yawed, global]"/1 -> left dx yawed/1
  Measurement Noise Covariance Matricies/1(R_no_position) -> "dX, ddX Kalman Filter"/5
  P0_kalman_transverse2/1 -> "dX, ddX Kalman Filter"/4
  Selector4/1 -> "dX, ddX Kalman Filter"/3
  Mux5/1 -> "dX, ddX Kalman Filter"/2
  right dx yawed/1 -> Mux5/2
  left dx yawed/1 -> Mux5/1
  eigen values1/1(E) -> "[y, dy, ddy] uncertainty"/1
  eigen values2/1(E) -> "[x, dx, ddx] uncertainty"/1
  Y State Kalman Filter/1 -> "[y, dy, ddy] [m/s, m/s^2]"/1
  y acceleration/1 -> Mux1/3
  x acceleration/1 -> Mux/3, Mux5/3
  z acceleration/1 -> Mux3/3
  COM XYZ Acceleration [m/s^2] x3/1 -> z acceleration/1, y acceleration/1, x acceleration/1
  Z State Kalman Filter/1 -> "[z, dz, ddz] [m, m/s, m/s^2]"/1
  GRFy [N]/1 -> Difference1/1
  Mux3/1 -> Z State Kalman Filter/2  "yawed [left z, right z, ddz]"
  GRFx [N]/1 -> Difference2/1
  Measurement Noise Covariance Matricies/3(R_vertical) -> Z State Kalman Filter/5
  Mux1/1 -> Y State Kalman Filter/2  "yawed [left y, right y, ddy]"
  Mux/1 -> X State Kalman Filter/2  "yawed [left x, right x, ddx]"
  Right Vertical GRF [N]/1 -> Measurement Noise Covariance Matricies/2(vertical_GRF_R)
  Left Vertical GRF [N]/1 -> Measurement Noise Covariance Matricies/1(vertical_GRF_L)
  "COM from Left Foot [body, yawed, global]"/1 -> left z yawed/1, left y yawed/1, left x yawed/1
  left x yawed/1 -> Mux/1
  "COM from Right Foot [body, yawed, global]"/1 -> right z yawed/1, right y yawed/1, right x yawed/1
  right x yawed/1 -> Mux/2
  left y yawed/1 -> Mux1/1
  right y yawed/1 -> Mux1/2
  left z yawed/1 -> Mux3/1
  right z yawed/1 -> Mux3/2
  "Initial [x, dx, ddx] [m, m/s, m/s^2]"/1 -> Selector4/1, X State Kalman Filter/3
  P0_kalman_transverse1/1 -> Y State Kalman Filter/4
  "Initial [y, dy, ddy] [m, m/s, m/s^2]"/1 -> Y State Kalman Filter/3
  "Initial [z, dz, ddz] [m m/s m/s^2]"/1 -> Z State Kalman Filter/3
  X State Kalman Filter/2 -> eigen values2/1(Z)
  Y State Kalman Filter/2 -> eigen values1/1(Z)
  Z State Kalman Filter/2 -> eigen values/1(Z)
  eigen values/1(E) -> "[z, dz, ddz] uncertainty"/1
  Logical Operator/1 -> Product/1, Product1/1, Product2/1
  Difference/1 -> Product/2
  Entering Stance [1/0]/1 -> Logical Operator/1, Y State Kalman Filter/5, X State Kalman Filter/5
  Difference1/1 -> Product1/2
  Difference2/1 -> Product2/2
  Product1/1 -> Y State Kalman Filter/1
  Product/1 -> Z State Kalman Filter/1
  GRFz [N]/1 -> Difference/1
  P0_kalman_transverse/1 -> X State Kalman Filter/4
  Product2/1 -> "dX, ddX Kalman Filter"/1, X State Kalman Filter/1
  X State Kalman Filter/1 -> Selector/1
  Selector/1 -> Mux2/1
  "dX, ddX Kalman Filter"/1 -> Mux2/2
  Mux2/1 -> "[x, dx, ddx] [m/s, m/s^2]"/1
  "dX, ddX Kalman Filter"/2 -> Terminator/1
  Measurement Noise Covariance Matricies/2(R_transverse) -> Y State Kalman Filter/6, X State Kalman Filter/6
  P0_kalman_vertical/1 -> Z State Kalman Filter/4

== system deadbeat_running_control/Behavior/State Estimation/Lowpass Filter ==
  In : Inport
  Generated Filter Block : dsparch4/Biquad Filter  Tag=BlockMethodSubSystem  IIRFiltStruct=Direct form II  CoeffSource=Specify via dialog  BiQuadCoeffs=[1.0218648663828083 -2 1.0218648663828083 1 -1.9114378222117407 0.91557643487411833]  a0Flag=Warning  IC=0  ICnum=0  ICden=0  denAccumFracLength=30  denProdOutputFracLength=30  secondMemoryFracLength=15  roundingMode=Floor  overflowMode=off  ScaleValues=[0.0041174265739107223;22.985401576126357]  optimizeScaleValues=off  ScaleValueMode=Specify via input port (g)  scaleValueFracLength=14  FilterSource=Specify via dialog  FilterObject=Hm_biquad
  Out : Outport
  wires:
  In/1 -> Generated Filter Block/1
  Generated Filter Block/1 -> Out/1

== system deadbeat_running_control/Behavior/Primary and Lateral Behavior/Circular Buffer (Left Foot)/Enabled on Touchdown ==
  In : Inport
  Enable : EnablePort
  Out : Outport
  wires:
  In/1 -> Out/1

== system deadbeat_running_control/Behavior/Primary and Lateral Behavior/Circular Buffer (Right Foot)/Enabled on Touchdown ==
  In : Inport
  Enable : EnablePort
  Out : Outport
  wires:
  In/1 -> Out/1

== system deadbeat_running_control/Behavior/Primary and Lateral Behavior/Flight/Back//Front PD ==
  Desired Position [rad] [back front] : Inport
  Desired Velocity [rad/s] [back front] : Inport  Port=2
  Measured Position [rad] [back front] : Inport  Port=3
  Measured Velocity [rad/s] [back front] : Inport  Port=4
  Back / Front Position Error : Scope  NumInputPorts=2
  Back / Front PositionTracking : Scope  NumInputPorts=2
  Demux : Demux  Outputs=2
  Feedback / Feedforward : Scope  NumInputPorts=2
  Kp_SEA_Trajectory : Constant  Value=kp_velocity_swing_trajectory
  Mux{1..2,12..13} (4 alike) : Mux  Inputs=2
  Primary Flight Back / Front Velocity Tracking : Scope  NumInputPorts=2
  Product1 : Product
  Selector{,1..3} (4 alike) : Selector  InputPortWidth=2  IndexOptions=Index vector (dialog)  Indices=[1]  OutputSizes=1
  Selector{4..5,7..8} (4 alike) : Selector  InputPortWidth=2  IndexOptions=Index vector (dialog)  Indices=[2]  OutputSizes=1
  Sum7 : Sum  Inputs=|+-
  Sum9 : Sum
  Commanded Velocity [rad/s] [back front] : Outport
  wires:
  Selector8/1 -> Mux12/2
  Selector7/1 -> Mux12/1
  Selector3/1 -> Mux1/2
  Selector2/1 -> Mux1/1
  Mux1/1 -> Primary Flight Back / Front Velocity Tracking/1
  Mux12/1 -> Primary Flight Back / Front Velocity Tracking/2
  Sum9/1 -> Commanded Velocity [rad/s] [back front]/1, Selector3/1, Selector8/1
  Measured Velocity [rad/s] [back front]/1 -> Selector2/1, Selector7/1
  Selector4/1 -> Mux2/1
  Selector5/1 -> Mux2/2
  Selector1/1 -> Mux13/2
  Selector/1 -> Mux13/1
  Mux2/1 -> Back / Front PositionTracking/2
  Desired Position [rad] [back front]/1 -> Sum7/1, Selector5/1, Selector1/1
  Mux13/1 -> Back / Front PositionTracking/1
  Measured Position [rad] [back front]/1 -> Selector/1, Selector4/1, Sum7/2
  Product1/1 -> Feedback / Feedforward/1, Sum9/1
  Kp_SEA_Trajectory/1 -> Product1/2
  Desired Velocity [rad/s] [back front]/1 -> Feedback / Feedforward/2, Sum9/2
  Sum7/1 -> Demux/1, Product1/1
  Demux/1 -> Back / Front Position Error/1
  Demux/2 -> Back / Front Position Error/2

== system deadbeat_running_control/Behavior/Primary and Lateral Behavior/Flight/Enabled Subsystem ==
  in : Inport
  Enable : EnablePort
  out : Outport
  wires:
  in/1 -> out/1

== system deadbeat_running_control/Behavior/Primary and Lateral Behavior/Flight/Hold Values on Takeoff ==
  in : Inport
  Trigger : TriggerPort  VariantControl=Variant  ShowOutputPort=on  PortDimensions=1
  Subsystem : Subsystem
  out : Outport
  wires:
  in/1 -> Subsystem/1(in)
  Subsystem/1(out) -> out/1
  Trigger/1 -> Subsystem/Enable

== system deadbeat_running_control/Behavior/Primary and Lateral Behavior/Hold Values on Takeoff/Subsystem ==
  in : Inport
  Enable : EnablePort
  out : Outport
  wires:
  in/1 -> out/1

== system deadbeat_running_control/Behavior/Primary and Lateral Behavior/Hold Values on Takeoff1/Subsystem ==
  in : Inport
  Enable : EnablePort
  out : Outport
  wires:
  in/1 -> out/1

== system deadbeat_running_control/Behavior/Primary and Lateral Behavior/Hold Values on Takeoff2/Subsystem ==
  in : Inport
  Enable : EnablePort
  out : Outport
  wires:
  in/1 -> out/1

== system deadbeat_running_control/Behavior/Primary and Lateral Behavior/Hold Values on Takeoff3/Subsystem ==
  in : Inport
  Enable : EnablePort
  out : Outport
  wires:
  in/1 -> out/1

== system deadbeat_running_control/Behavior/Primary and Lateral Behavior/Stance/2D Inverse Dynamics ==
  Fx Desired [N] : Inport
  Fz Desired [N] : Inport  Port=2
  Leg Length [m m/s] : Inport  Port=3
  Leg Angle [rad rad/s] : Inport  Port=4
  Torso Pitch [rad rad/s] : Inport  Port=5
  Primary w [m] : Inport  Port=6
  Constant2 : Constant  Value=0
  Demux5 : Demux  Outputs=2
  Leg Force-Torque Distribution : Subsystem
  Spring Torques : Selector  InputPortWidth=7  IndexOptions=Index vector (dialog)  Indices=[6 7]  OutputSizes=1
  target_GRF_inverse_dynamics : MATLAB Function  TreatAsAtomicUnit=on
  Leg Torque [Nm] : Outport
  Leg Force [N] : Outport  Port=2
  wires:
  Leg Force-Torque Distribution/1(Leg Force [N]) -> Leg Force [N]/1
  Leg Angle [rad rad/s]/1 -> target_GRF_inverse_dynamics/4(phi)
  Torso Pitch [rad rad/s]/1 -> target_GRF_inverse_dynamics/3(theta)
  Leg Force-Torque Distribution/2(Leg Torque [Nm]) -> Leg Torque [Nm]/1
  Primary w [m]/1 -> target_GRF_inverse_dynamics/6(w), Leg Force-Torque Distribution/3(w [m])
  Spring Torques/1 -> Demux5/1
  Demux5/1 -> Leg Force-Torque Distribution/1(Front Spring Torque [Nm])
  Demux5/2 -> Leg Force-Torque Distribution/2(Back Spring Torque [Nm])
  target_GRF_inverse_dynamics/1(z) -> Spring Torques/1
  Constant2/1 -> target_GRF_inverse_dynamics/8(tau_rotor_b), target_GRF_inverse_dynamics/7(tau_rotor_f)
  Leg Length [m m/s]/1 -> target_GRF_inverse_dynamics/5(l_leg)
  Fx Desired [N]/1 -> target_GRF_inverse_dynamics/1(GRFx)
  Fz Desired [N]/1 -> target_GRF_inverse_dynamics/2(GRFz)

== system deadbeat_running_control/Behavior/Primary and Lateral Behavior/Stance/Chirp Frequency ==
  Time Since Stance : Inport
  Chirp Freq Factor Saturation : Saturate  UpperLimit=standing_bounce_max_chirp_scale  LowerLimit=0
      settings: AttributesFormatString=Top: %<UpperLimit>\nBottom: %<LowerLimit>
  Compare To Constant1 : simulink/Logic and Bit Operations/Compare To Constant  relop=~=  const=standing_bounce_max_chirp_scale  OutDataTypeStr=boolean
  Constant1 : Constant
  Constant5 : Constant  Value=standing_bounce_increase_rate
  Product{1..4} (4 alike) : Product
  Sum : Sum  Inputs=++|
  standing_bounce_frequency : Constant  Value=standing_bounce_frequency
  w : Outport
  dw/dt : Outport  Port=2
  wires:
  standing_bounce_frequency/1 -> Product2/1, Product3/1
  Chirp Freq Factor Saturation/1 -> Product3/2, Compare To Constant1/1
  Product3/1 -> w/1
  Product1/1 -> dw/dt/1
  Compare To Constant1/1 -> Product1/1
  Product2/1 -> Product1/2
  Constant5/1 -> Product2/2, Product4/2
  Time Since Stance/1 -> Product4/1
  Sum/1 -> Chirp Freq Factor Saturation/1
  Product4/1 -> Sum/2
  Constant1/1 -> Sum/1

== system deadbeat_running_control/Behavior/Primary and Lateral Behavior/Stance/Compute Forces1 ==
  XYZ Acceleration : Inport
  Constant5 : Constant  Value=g
  Demux : Demux  Outputs=3
  Gain4 : Gain  Gain=m_total_real
  Mux : Mux  Inputs=3
  Sum8 : Sum  Inputs=|++
  XYZ Force : Outport
  wires:
  Constant5/1 -> Sum8/2
  XYZ Acceleration/1 -> Demux/1
  Gain4/1 -> XYZ Force/1
  Mux/1 -> Gain4/1
  Sum8/1 -> Mux/3
  Demux/3 -> Sum8/1
  Demux/2 -> Mux/2
  Demux/1 -> Mux/1

== system deadbeat_running_control/Behavior/Primary and Lateral Behavior/Stance/Hold Values on Takeoff ==
  in : Inport
  Trigger : TriggerPort  VariantControl=Variant  ShowOutputPort=on  PortDimensions=1
  Subsystem : Subsystem
  out : Outport
  wires:
  Trigger/1 -> Subsystem/Enable
  Subsystem/1(out) -> out/1
  in/1 -> Subsystem/1(in)

== system deadbeat_running_control/Behavior/Primary and Lateral Behavior/Stance/Hold Values on Touchdown ==
  in : Inport
  Trigger : TriggerPort  VariantControl=Variant  ShowOutputPort=on  PortDimensions=1
  Subsystem : Subsystem
  out : Outport
  wires:
  in/1 -> Subsystem/1(in)
  Subsystem/1(out) -> out/1
  Trigger/1 -> Subsystem/Enable

== system deadbeat_running_control/Behavior/Primary and Lateral Behavior/Stance/Lowpass Filter ==
  In : Inport
  Generated Filter Block : dsparch4/Biquad Filter  Tag=BlockMethodSubSystem  IIRFiltStruct=Direct form II  CoeffSource=Specify via dialog  BiQuadCoeffs=[1.2169083457291219 -2 1.2169083457291219 1 -1.7334293610249598 0.76768521888208641]  a0Flag=Warning  IC=0  ICnum=0  ICden=0  denAccumFracLength=30  denProdOutputFracLength=30  secondMemoryFracLength=15  roundingMode=Floor  overflowMode=off  ScaleValues=[0.034049223021428709;2.3191101889079508]  optimizeScaleValues=off  ScaleValueMode=Specify via input port (g)  scaleValueFracLength=14  FilterSource=Specify via dialog  FilterObject=Hm_biquad
  Out : Outport
  wires:
  In/1 -> Generated Filter Block/1
  Generated Filter Block/1 -> Out/1

== system deadbeat_running_control/Behavior/Primary and Lateral Behavior/Stance/Torque Distribution ==
  Leg Torque [Nm] : Inport
  Leg Force [N] : Inport  Port=2
  w [m] : Inport  Port=3
  Gain : Gain  Gain=0.5
  Gain1 : Gain  Gain=0.5
  Motor Torque Saturation Optimization : MATLAB Function  Commented=on  TreatAsAtomicUnit=on
  Primary Front Back Torque : Scope  NumInputPorts=2
  Product : Product  RndMeth=Zero
  Sum : Sum  Inputs=|++
  Sum1 : Sum  Inputs=+-|
  Back Torque [Nm] : Outport
  Front Torque [Nm] : Outport  Port=2
  wires:
  Product/1 -> Gain1/1
  Leg Force [N]/1 -> Product/1
  Gain1/1 -> Sum/2, Sum1/2
  w [m]/1 -> Product/2
  Gain/1 -> Sum1/1, Sum/1
  Sum/1 -> Primary Front Back Torque/1, Front Torque [Nm]/1
  Leg Torque [Nm]/1 -> Gain/1
  Sum1/1 -> Primary Front Back Torque/2, Back Torque [Nm]/1

== system deadbeat_running_control/Behavior/Primary and Lateral Behavior/Flight/Hold Values on Takeoff/Subsystem ==
  in : Inport
  Enable : EnablePort
  out : Outport
  wires:
  in/1 -> out/1

== system deadbeat_running_control/Behavior/Primary and Lateral Behavior/Stance/2D Inverse Dynamics/Leg Force-Torque Distribution ==
  Front Spring Torque [Nm] : Inport
  Back Spring Torque [Nm] : Inport  Port=2
  w [m] : Inport  Port=3
  Divide : Product  Inputs=*/
  Sum2 : Sum  Inputs=+|+
  Sum5 : Sum  Inputs=+|-
  Leg Force [N] : Outport
  Leg Torque [Nm] : Outport  Port=2
  wires:
  Sum2/1 -> Leg Torque [Nm]/1
  Back Spring Torque [Nm]/1 -> Sum5/2, Sum2/2
  Sum5/1 -> Divide/1
  w [m]/1 -> Divide/2
  Front Spring Torque [Nm]/1 -> Sum5/1, Sum2/1
  Divide/1 -> Leg Force [N]/1

== system deadbeat_running_control/Behavior/Primary and Lateral Behavior/Stance/Hold Values on Takeoff/Subsystem ==
  in : Inport
  Enable : EnablePort
  out : Outport
  wires:
  in/1 -> out/1

== system deadbeat_running_control/Behavior/Primary and Lateral Behavior/Stance/Hold Values on Touchdown/Subsystem ==
  in : Inport
  Enable : EnablePort
  out : Outport
  wires:
  in/1 -> out/1

== matlab function deadbeat_running_control/Behavior/Compute World Frame COM Coordinates from Yawed Frame ==
  data: com_position_world output; X_dX input; Y_dY input; Z_dZ input; torso_yaw input; com_velocity_world output
function [com_position_world, com_velocity_world] ...
          = compute_com_state_in_world_frame(X_dX, Y_dY, Z_dZ, torso_yaw)

    R_yawed_to_world = R_yaw(torso_yaw(1));
    dR_yawed_to_world = dR_yaw(torso_yaw(1),torso_yaw(2));
    
    com_position_yawed = [X_dX(1); Y_dY(1); Z_dZ(1)];
    com_velocity_yawed = [X_dX(2); Y_dY(2); Z_dZ(2)];
    
    com_position_world = R_yawed_to_world*com_position_yawed;
    com_velocity_world = dR_yawed_to_world*com_position_yawed + R_yawed_to_world*com_velocity_yawed;

end

function R_gy = R_yaw(psi) % map yawed frame to global
  R_gy = [cos(psi), -sin(psi), 0; sin(psi), cos(psi), 0; 0 0 1]; 
end
function dR_gy = dR_yaw(psi,dpsi)
  dR_gy = dpsi*[-sin(psi), -cos(psi), 0; cos(psi), -sin(psi), 0; 0 0 0];
end
